simulink model "Arduino33IotNano"  (R2022b)
settings: Solver=FixedStepAuto  StartTime=0.0  StopTime=inf  RelTol=1e-3  EnableMultiTasking=on
values from neighbouring files (symbols this model uses):
  Ts = 0.01    [RegulatorLiniarizare2.m]
libraries: arduinomotorcarrierlib x3, simulink x1, eeGeneralControl x1, arduinosensorlib x1
settings Model: SimulationMode=external  ExtModeTrigDuration=2  Creator=tudorn  LastModifiedBy=tudorn
settings OptimizationCC: EnhancedBackFolding=on  PassReuseOutputArgsAs=Individual arguments  ZeroExternalMemoryAtStartup=off  ZeroInternalMemoryAtStartup=off  MaxStackSize=64  OptimizeBlockOrder=speed  DifferentSizesBufferReuse=on  OptimizationCustomize=off  EfficientTunableParamExpr=on
settings DebuggingCC: ParameterTunabilityLossMsg=error
settings HardwareCC: ProdBitPerPointer=32  ProdBitPerSizeT=32  ProdBitPerPtrDiffT=32  ProdLargestAtomicInteger=Long  ProdLargestAtomicFloat=Double  ProdWordSize=32  ProdHWDeviceType=ARM Compatible->ARM Cortex  UseEmbeddedCoderFeatures=off  UseSimulinkCoderFeatures=off
settings SFSimCC: MATLABDynamicMemAlloc=off
settings RTWCC: Description=Embedded Coder  SystemTargetFile=ert.tlc  HardwareBoard=Arduino Nano 33 IoT  TemplateMakefile=ert_default_tmf  RTWVerbose=off  Toolchain=Arduino ARM  BuildConfiguration=Faster Runs
settings CodeAppCC: ForceParamTrailComments=on  OperatorAnnotations=on  SimulinkDataObjDesc=on  SFDataObjDesc=on  MangleLength=10  InsertBlockDesc=on
settings ERTTargetCC: SupportContinuousTime=on  SupportNonInlinedSFcns=on  SupportVariableSizeSignals=on  ExtMode=on  ExtModeTransport=3  ExtModeStaticAlloc=on  ExtModeAutomaticAllocSize=off  ExtModeStaticAllocSize=8192  ExtModeMexFile=ext_xcp  ExtModeMexArgs=0 '/dev/cu.usbmodem101' 115200  ExtModeIntrfLevel=Level2 - Open  ERTSrcFileBannerTemplate=codertarget_code_template.cgt  ERTHdrFileBannerTemplate=codertarget_code_template.cgt  ERTDataSrcFileTemplate=codertarget_code_template.cgt  ERTDataHdrFileTemplate=codertarget_code_template.cgt

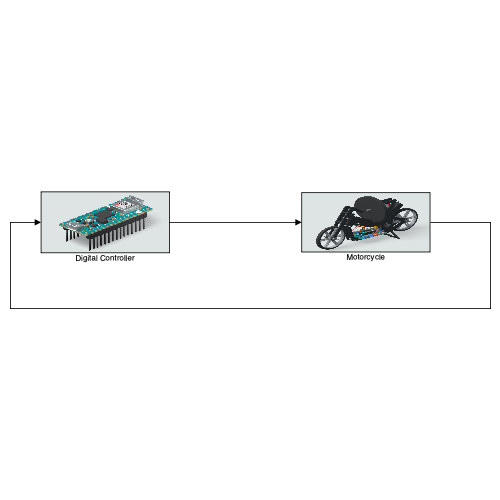
[thumbnail: Simulink's stored preview of the top-level diagram]
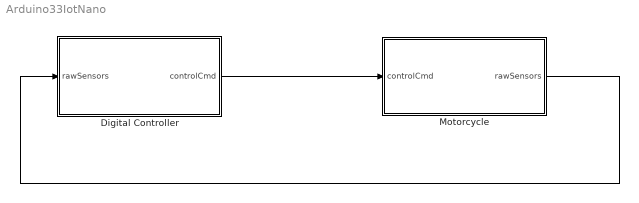
== system Arduino33IotNano ==
  Digital Controller : Subsystem
      mask Display: image('arduinoNano.jpg'); % Use "Edit Image" on toolstrip to change.
  Motorcycle : Subsystem
      mask Display: image('motorcycle.png'); % Use "Edit Image" on toolstrip to change.
  wires:
  Digital Controller/1(controlCmd) -> Motorcycle/1(controlCmd)
  Motorcycle/1(rawSensors) -> Digital Controller/1(rawSensors)

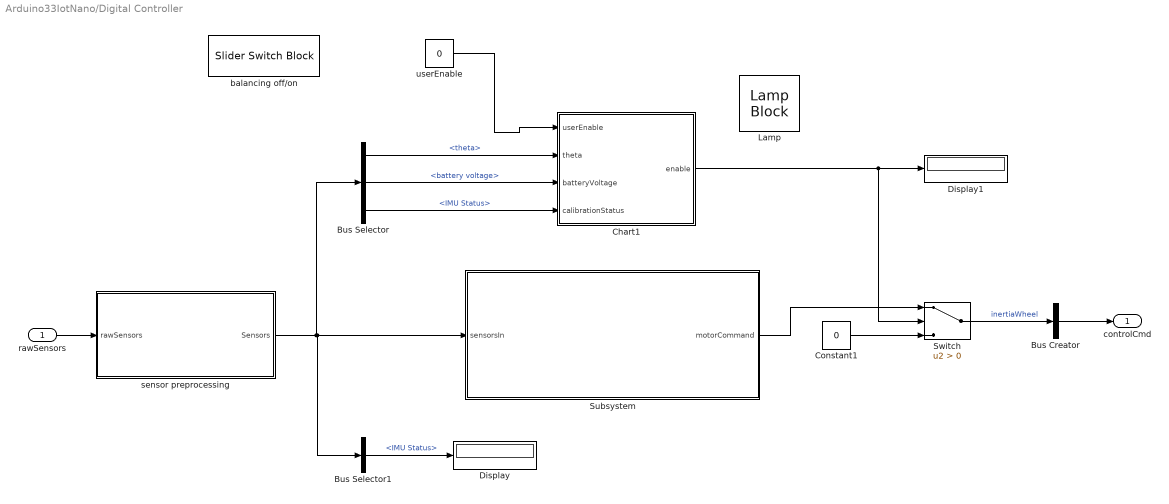
== system Arduino33IotNano/Digital Controller ==
  rawSensors : Inport
  Bus Creator : BusCreator  Inputs=1
  Bus Selector : BusSelector  OutputSignals=theta,battery voltage,IMU Status
  Bus Selector1 : BusSelector  OutputSignals=IMU Status
  Chart1 : Stateflow chart  TreatAsAtomicUnit=on
  Constant1 : Constant  Value=0  SampleTime=Ts
  Display : Display
  Display1 : Display
  Lamp : LampBlock  LabelPosition=Hide
  Subsystem : Subsystem
  Switch : Switch  Criteria=u2 > Threshold  SaturateOnIntegerOverflow=off  InputSameDT=off
  balancing off/on : SliderSwitchBlock  LabelPosition=Bottom
      settings: Values={{'Off', 'On'}, [0 1]}
  sensor preprocessing : Subsystem
  userEnable : Constant  Value=0  SampleTime=Ts
  controlCmd : Outport
  wires:
  Bus Creator/1 -> controlCmd/1
  Switch/1 -> Bus Creator/1  "inertiaWheel"
  rawSensors/1 -> sensor preprocessing/1(rawSensors)
  Bus Selector/1 -> Chart1/2(theta)  "<theta>"
  Chart1/1(enable) -> Display1/1, Switch/2
  Constant1/1 -> Switch/3
  userEnable/1 -> Chart1/1(userEnable)
  Bus Selector/2 -> Chart1/3(batteryVoltage)  "<battery voltage>"
  Bus Selector/3 -> Chart1/4(calibrationStatus)  "<IMU Status>"
  sensor preprocessing/1(Sensors) -> Bus Selector1/1, Subsystem/1(sensorsIn), Bus Selector/1
  Subsystem/1(motorCommand) -> Switch/1
  Bus Selector1/1 -> Display/1  "<IMU Status>"

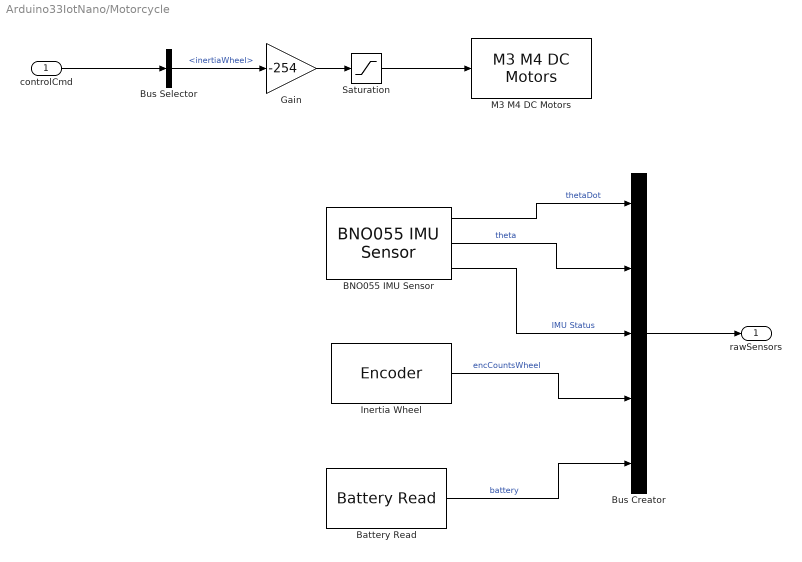
== system Arduino33IotNano/Motorcycle ==
  controlCmd : Inport
  BNO055 IMU Sensor : arduinosensorlib/BNO055 IMU Sensor  SlaveAddress=0x28  OperationMode=Fusion  Accel=off  AngularRate=on  MagField=off  EulerAngles=on  Quat=off  LinearAccel=off  GravityVector=off  Status=on  Timestamp=off  AccelRange=4G  AccelBW=62.5 Hz  GyroRange=2000 dps  GyroBW=32 Hz  MagODR=10 Hz  spf=1  SampleTime=0.01  blockPlatform=ARDUINO  QueueSizeFactor=1
  Battery Read : arduinomotorcarrierlib/Battery Read  SlaveAddress=uint8( hex2dec( '66' ) )  blockPlatform=ARDUINO  SampleTime=Ts
  Bus Creator : BusCreator  Inputs=5
  Bus Selector : BusSelector  OutputSignals=inertiaWheel
  Gain : Gain  Gain=-254
  Inertia Wheel : arduinomotorcarrierlib/Encoder  SlaveAddress=uint8( hex2dec( '66' ) )  blockPlatform=ARDUINO  Encoder=1  ShowSpeed=off  ResetOption=on  SampleTime=Ts
  M3 M4 DC Motors : arduinomotorcarrierlib/M3 M4 DC Motors  MotorNumber=M3  forwardPinNumber=3  reversePinNumber=2
  Saturation : Saturate  UpperLimit=255  LowerLimit=-255
  rawSensors : Outport
  wires:
  BNO055 IMU Sensor/1 -> Bus Creator/1  "thetaDot"
  BNO055 IMU Sensor/2 -> Bus Creator/2  "theta"
  BNO055 IMU Sensor/3 -> Bus Creator/3  "IMU Status"
  Inertia Wheel/1 -> Bus Creator/4  "encCountsWheel"
  Battery Read/1 -> Bus Creator/5  "battery"
  Bus Creator/1 -> rawSensors/1
  controlCmd/1 -> Bus Selector/1
  Bus Selector/1 -> Gain/1  "<inertiaWheel>"
  Gain/1 -> Saturation/1
  Saturation/1 -> M3 M4 DC Motors/1

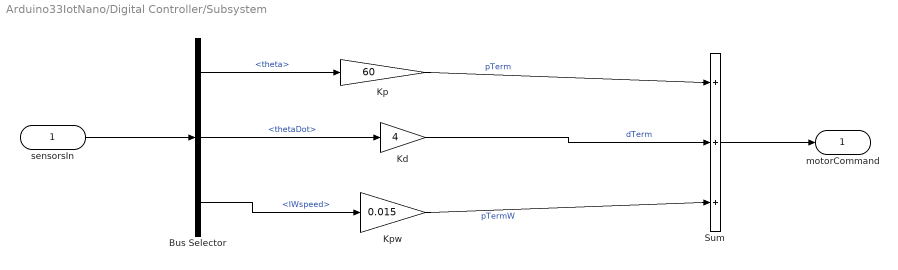
== system Arduino33IotNano/Digital Controller/Subsystem ==
  sensorsIn : Inport
  Bus Selector : BusSelector  OutputSignals=theta,thetaDot,IWspeed
  Kd : Gain  Gain=4
  Kp : Gain  Gain=60
  Kpw : Gain  Gain=0.015
  Sum : Sum  Inputs=+|+|+
  motorCommand : Outport
  wires:
  sensorsIn/1 -> Bus Selector/1
  Bus Selector/3 -> Kpw/1  "<IWspeed>"
  Bus Selector/2 -> Kd/1  "<thetaDot>"
  Bus Selector/1 -> Kp/1  "<theta>"
  Sum/1 -> motorCommand/1
  Kp/1 -> Sum/1  "pTerm"
  Kd/1 -> Sum/2  "dTerm"
  Kpw/1 -> Sum/3  "pTermW"

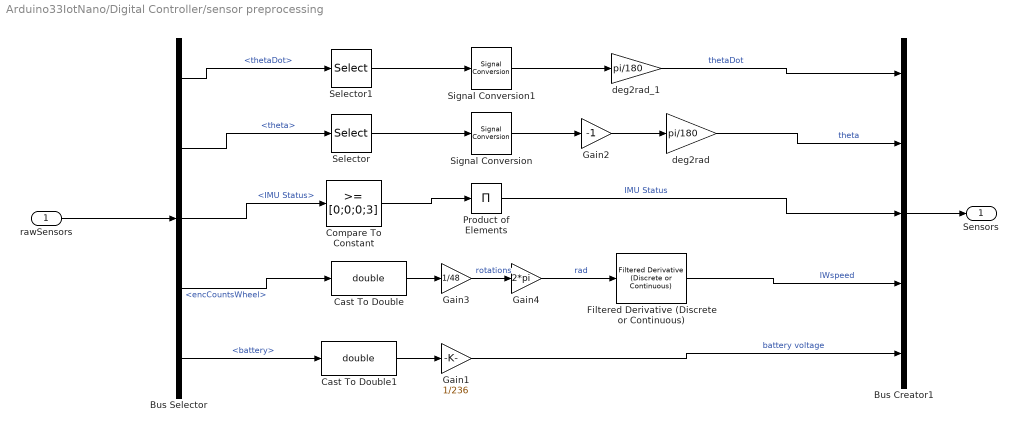
== system Arduino33IotNano/Digital Controller/sensor preprocessing ==
  rawSensors : Inport
  Bus Creator1 : BusCreator  Inputs=5
  Bus Selector : BusSelector  OutputSignals=thetaDot,theta,IMU Status,encCountsWheel,battery
  Cast To Double : DataTypeConversion  OutDataTypeStr=double  SaturateOnIntegerOverflow=off  RndMeth=Floor
  Cast To Double1 : DataTypeConversion  OutDataTypeStr=double  SaturateOnIntegerOverflow=off  RndMeth=Floor
  Compare To Constant : simulink/Logic and Bit Operations/Compare To Constant  relop=>=  const=[0;0;0;3]  OutDataTypeStr=boolean
  Filtered Derivative (Discrete or Continuous) : eeGeneralControl/Filtered Derivative (Discrete or Continuous)  K=1  T=0.1  B=inf  A=-inf  minRatio=10  init_option=Inherited from block input  x0=0  Ts=-1
      settings: LibrarySourceBlock=|
      | ee_sl_lib/General Control/Filtered Derivative
      | (Discrete or Continuous)
  Gain1 : Gain  Gain=1/236
  Gain2 : Gain  Gain=-1
  Gain3 : Gain  Gain=1/48
  Gain4 : Gain  Gain=2*pi
  Product of Elements : Product  Inputs=*
  Selector : Selector  InputPortWidth=3  IndexOptions=Index vector (dialog)  Indices=[2]  OutputSizes=1
  Selector1 : Selector  InputPortWidth=3  IndexOptions=Index vector (dialog)  Indices=[2]  OutputSizes=1
  Signal Conversion : SignalConversion  OverrideOpt=off
  Signal Conversion1 : SignalConversion  OverrideOpt=off
  deg2rad : Gain  Gain=pi/180
  deg2rad_1 : Gain  Gain=pi/180
  Sensors : Outport
  wires:
  deg2rad/1 -> Bus Creator1/2  "theta"
  Gain2/1 -> deg2rad/1
  deg2rad_1/1 -> Bus Creator1/1  "thetaDot"
  Bus Selector/5 -> Cast To Double1/1  "<battery>"
  Filtered Derivative (Discrete or Continuous)/1 -> Bus Creator1/4  "IWspeed"
  Gain4/1 -> Filtered Derivative (Discrete or Continuous)/1  "rad"
  Cast To Double1/1 -> Gain1/1
  Selector/1 -> Signal Conversion/1
  Bus Creator1/1 -> Sensors/1
  Product of Elements/1 -> Bus Creator1/3  "IMU Status"
  Signal Conversion1/1 -> deg2rad_1/1
  Cast To Double/1 -> Gain3/1
  Gain3/1 -> Gain4/1  "rotations"
  Bus Selector/2 -> Selector/1  "<theta>"
  rawSensors/1 -> Bus Selector/1
  Compare To Constant/1 -> Product of Elements/1
  Signal Conversion/1 -> Gain2/1
  Selector1/1 -> Signal Conversion1/1
  Bus Selector/4 -> Cast To Double/1  "<encCountsWheel>"
  Gain1/1 -> Bus Creator1/5  "battery voltage"
  Bus Selector/3 -> Compare To Constant/1  "<IMU Status>"
  Bus Selector/1 -> Selector1/1  "<thetaDot>"

== stateflow chart Arduino33IotNano/Digital Controller/Chart1 ==
  state checkFallen [parallel]
    settings: executionOrder=1
    state fallen
      entry: upright = false
    state standing
      entry: upright = true
    (default) -> fallen
    fallen -> standing : [abs(theta) <pi*8/180]
    standing -> fallen : [abs(theta) > pi*8/180]
  state checkIMUCalib [parallel]
    settings: executionOrder=2
    state imuNotCalibrated
      entry:
      IMUCalibrated = false;
    state imuCalibrated
      entry:
      IMUCalibrated = true;
    (default) -> imuNotCalibrated
    imuNotCalibrated -> imuCalibrated : [calibrationStatus == true]
  state checkBattery [parallel]
    settings: executionOrder=3
    state batteryNotCharged
      entry:
      batteryOK = false;
    state batteryCharged
      entry:
      batteryOK = true;
    (default) -> batteryNotCharged
    batteryCharged -> batteryNotCharged : [batteryVoltage < 3.7]
    batteryNotCharged -> batteryCharged : [batteryVoltage >= 3.7]
  state calculateEnable [parallel]
    settings: executionOrder=4
    state disableControl
      entry: enable = false
    state enableControl
      entry: enable = true
    (default) -> disableControl
    disableControl -> enableControl : [userEnable&& batteryOK && IMUCalibrated && upright]
    enableControl -> disableControl : [not(userEnable) || not(batteryOK) || not(IMUCalibrated) || not(upright)]
  data: userEnable input; theta input; enable output; batteryVoltage input; calibrationStatus input; upright local; IMUCalibrated local; batteryOK local
